simulink model "simulation_darko_vol_ligne"  (R2021b)
settings: Solver=ode23s  StartTime=0.0  StopTime=60  FixedStep=0.0001  MaxStep=1e-2  RelTol=1e-3
values from neighbouring files (symbols this model uses):
  controlleur = struct('k1',1.0,                       'kc',5,                       'kv',1.0,                       'ku',600.0,                       'kgamma',1.0,                       'M_k',M_k,                       'kd',60,                       'k_s',0.01                       )    [generateContolleur.m]    (also in run_vol_ligne.m = generateContolleur(drone))
  drone = generateDarko()    [jacobian.m]    (also in run_vol_ligne.m)
  initial_state = [p_initial; v_initial; q_initial; omega_initial]    [run_vol_ligne.m]
  p2 = [1000; 1000; 1000]    [run_vol_ligne.m]
  speed = 20    [run_vol_ligne.m]
libraries: simulink_extras x6, aerolibanim x1, slpidlib x1, sharedtransform x1
settings Model: Creator=florian  LastModifiedBy=florian
settings SolverCC: AlgebraicLoopSolver=TrustRegion
settings DebuggingCC: SFMachineParentedDataDiag=warning

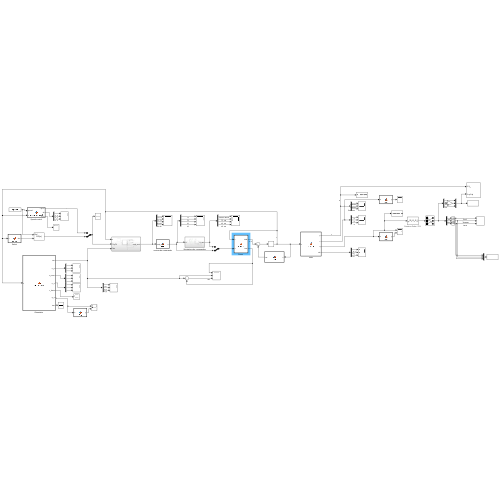
[thumbnail: Simulink's stored preview of the top-level diagram]
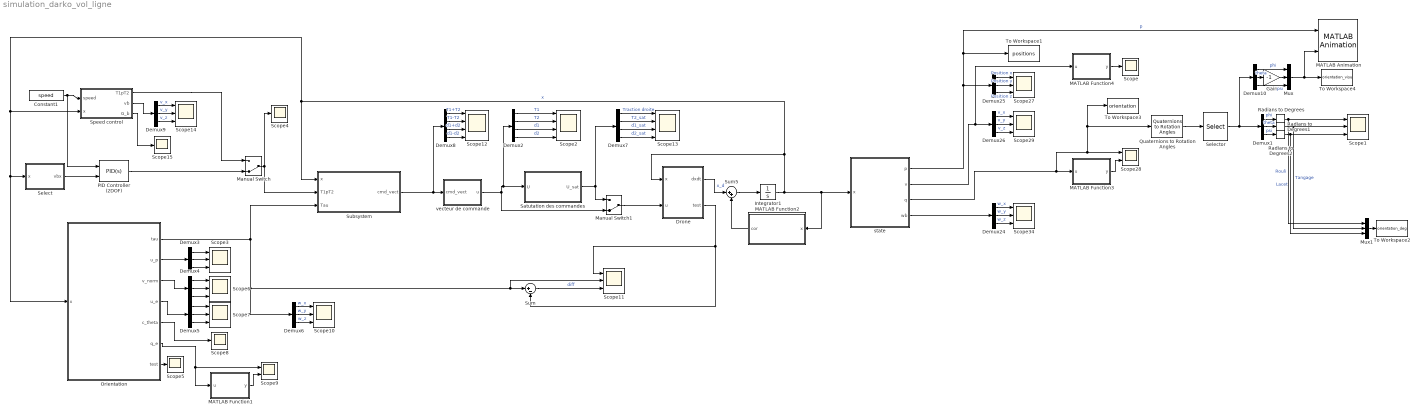
== system simulation_darko_vol_ligne ==
  Constant1 : Constant  Value=speed
  Demux{1,3..6,9..10,24..26} (10 alike) : Demux  Outputs=3
  Demux2 : Demux
  Demux7 : Demux
  Demux8 : Demux
  Drone : MATLAB Function  TreatAsAtomicUnit=on
  Gain : Gain  Gain=-1
  Integrator1 : Integrator  InitialCondition=initial_state
  MATLAB Animation : aerolibanim/MATLAB Animation  Tag=Matlab Animation 6 DOF  Vehicles=1  Geometries='astredwedge.mat'  BoundingBoxCoordinates=[-50,50,-50,50,-50,50]  CameraOffset=[-150,-50,0]  CameraViewAngle=3  SampleTime=0.2  FigurePosition=[962,411,639,384]
      settings: SourceProductBaseCode=AE
  MATLAB Function1 : MATLAB Function  TreatAsAtomicUnit=on
  MATLAB Function2 : MATLAB Function  TreatAsAtomicUnit=on
  MATLAB Function3 : MATLAB Function  TreatAsAtomicUnit=on
  MATLAB Function4 : MATLAB Function  TreatAsAtomicUnit=on
  Manual Switch : ManualSwitch  CurrentSetting=0
  Manual Switch1 : ManualSwitch  CurrentSetting=0
  Mux : Mux  Inputs=3
  Mux1 : Mux  Inputs=3
  Orientation : MATLAB Function  TreatAsAtomicUnit=on
  PID Controller (2DOF) : slpidlib/PID Controller (2DOF)  Controller=PID  Form=Parallel  TimeDomain=Continuous-time  UseExternalTs=off  SampleTime=-1  IntegratorMethod=Forward Euler  FilterMethod=Forward Euler  ControllerParametersSource=internal  P=1  I=1  D=0.1  UseFilter=on  N=100  b=1  c=1  TunerSelectOption=Transfer Function Based (PID Tuner App)  InitialConditionSource=internal  InitialConditionForIntegrator=0  InitialConditionForFilter=0  DifferentiatorICPrevScaledInput=0  ExternalReset=none  TrackingMode=off  Kt=1  LimitOutput=off  SatLimitsSource=internal  UpperSaturationLimit=inf  LowerSaturationLimit=-inf  LinearizeAsGain=on  AntiWindupMode=none  Kb=1  POutMin=[]  POutMax=[]  IOutMin=[]  IOutMax=[]  DOutMin=[]  DOutMax=[]  NOutMin=[]  NOutMax=[]  bOutMin=[]  bOutMax=[]  cOutMin=[]  cOutMax=[]  SumOutMin=[]  SumOutMax=[]  SaturationOutMin=[]  SaturationOutMax=[]  PParamMin=[]  PParamMax=[]  IParamMin=[]  IParamMax=[]  DParamMin=[]  DParamMax=[]  NParamMin=[]  NParamMax=[]  bParamMin=[]  bParamMax=[]  cParamMin=[]  cParamMax=[]  KbParamMin=[]  KbParamMax=[]  KtParamMin=[]  KtParamMax=[]  KbOutMin=[]  KbOutMax=[]  KtOutMin=[]  KtOutMax=[]  IntegratorOutMin=[]  IntegratorOutMax=[]  FilterOutMin=[]  FilterOutMax=[]  SumI1OutMin=[]  SumI1OutMax=[]  SumI2OutMin=[]  SumI2OutMax=[]  SumI3OutMin=[]  SumI3OutMax=[]  SumI4OutMin=[]  SumI4OutMax=[]  SumDOutMin=[]  SumDOutMax=[]  Sum1OutMin=[]  Sum1OutMax=[]  Sum2OutMin=[]  Sum2OutMax=[]  Sum3OutMin=[]  Sum3OutMax=[]  DifferentiatorOutMin=[]  DifferentiatorOutMax=[]  FilterDiffOutCoefMin=[]  FilterDiffOutCoefMax=[]  ReciprocalOutMin=[]  ReciprocalOutMax=[]  SumDenOutMin=[]  SumDenOutMax=[]  SumNumOutMin=[]  SumNumOutMax=[]  DivideOutMin=[]  DivideOutMax=[]  UdiffTsProdOutMin=[]  UdiffTsProdOutMax=[]  NTsProdOutMin=[]  NTsProdOutMax=[]  UintegralTsProdOutMin=[]  UintegralTsProdOutMax=[]  UngainTsProdOutMin=[]  UngainTsProdOutMax=[]  IntegratorContinuousStateAttributes=''  IntegratorStateMustResolveToSignalObject=off  IntegratorRTWStateStorageClass=Auto  FilterContinuousStateAttributes=''  FilterStateMustResolveToSignalObject=off  FilterRTWStateStorageClass=Auto  ParallelPVariant=InternalParameters  IdealPVariant=Disabled  IVariant=InternalParameters  DVariant=InternalParameters  bVariant=InternalParameters  cVariant=InternalParameters  IntegratorVariant=Continuous  SatVariant=Disabled  AWVariant=Passthrough  PCopyVariant=Disabled  TRVariant=Disabled  FdbkBlocksVariant=Forward  IdealPFdbkVariant=Disabled  SatFdbkVariant=Disabled  DerivativeFilterVariant=ContFilter  NVariant=InternalParameters  NCopyVariant=Disabled  FilterICVariant=InternalICsFilter  IntegratorICVariant=InternalICs  ExternalResetVariant=Disabled  TRSumVariant=Passthrough  SumFdbkVariant=Disabled  SumVariant=Sum_PID  TsampFilterVariant=InternalTs  TsampNgainVariant=Passthrough  TsampIntegralVariant=Passthrough  ExternalSaturationOutDataTypeStr=Inherit: Same as second input
      settings: SourceProductBaseCode=SL
  Quaternions to Rotation Angles : sharedtransform/Quaternions to Rotation Angles  rotationOrder=ZXY  aMode=aMode
      settings: SourceProductBaseCode=AE,PW,DR,MT,UV,VE
  Radians to Degrees : simulink_extras/Transformations/Radians to Degrees
  Radians to Degrees1 : simulink_extras/Transformations/Radians to Degrees
  Radians to Degrees2 : simulink_extras/Transformations/Radians to Degrees
  Satutation des commandes : Subsystem
  Scope{,4..5,8,15} (5 alike) : Scope
  Scope{1,3,6..7,10..11,14,27,29,34} (10 alike) : Scope  NumInputPorts=3
  Scope12 : Scope  NumInputPorts=4
  Scope13 : Scope  NumInputPorts=4
  Scope2 : Scope  NumInputPorts=4
  Scope28 : Scope  NumInputPorts=2
  Scope9 : Scope  NumInputPorts=2
  Select : MATLAB Function  TreatAsAtomicUnit=on
  Selector : Selector  InputPortWidth=3  IndexOptions=Index vector (dialog)  Indices=[2 3 1]  OutputSizes=1
  Speed control : MATLAB Function  TreatAsAtomicUnit=on
  Subsystem : Subsystem
  Sum : Sum  Inputs=|+-
  Sum5 : Sum  Inputs=|++
  To Workspace1 : ToWorkspace  VariableName=positions  SampleTime=-1
  To Workspace2 : ToWorkspace  VariableName=orientation_deg  SampleTime=-1
  To Workspace3 : ToWorkspace  VariableName=orientation  SampleTime=-1
  To Workspace4 : ToWorkspace  VariableName=orientation_visu  SampleTime=-1
  state : MATLAB Function  TreatAsAtomicUnit=on
  vecteur de commande : MATLAB Function  TreatAsAtomicUnit=on
  wires:
  Demux24/1 -> Scope34/1  "w_x"
  MATLAB Function3/1(y) -> Scope28/2
  Drone/1(dxdt) -> Sum5/1  "x_d"
  Demux24/2 -> Scope34/2  "w_y"
  Demux25/2 -> Scope27/2  "Position y"
  Integrator1/1 -> Drone/1(x), Select/1(x), Orientation/1(x), Speed control/2(x), Subsystem/1(x), MATLAB Function2/1(x), state/1(x)  "x"
  state/3(q) -> Scope28/1, To Workspace3/1, Quaternions to Rotation Angles/1, MATLAB Function3/1(u)
  Sum5/1 -> Integrator1/1
  MATLAB Function2/1(cor) -> Sum5/2
  Demux26/3 -> Scope29/3  "v_z"
  Demux26/2 -> Scope29/2  "v_y"
  Demux25/1 -> Scope27/1  "Position x"
  Demux25/3 -> Scope27/3  "Position z"
  state/1(p) -> MATLAB Animation/1, To Workspace1/1, Demux25/1  "p"
  Demux24/3 -> Scope34/3  "w_z"
  Demux26/1 -> Scope29/1  "v_x"
  Quaternions to Rotation Angles/1 -> Selector/1
  Satutation des commandes/1(U_sat) -> Demux7/1, Manual Switch1/1
  state/2(v) -> MATLAB Function4/1(u), Demux26/1
  Constant1/1 -> PID Controller (2DOF)/1, Speed control/1(speed)
  state/4(wb) -> Demux24/1
  Demux1/3 -> Radians to Degrees2/1  "psi"
  Demux1/2 -> Radians to Degrees1/1  "theta"
  Demux1/1 -> Radians to Degrees/1  "phi"
  Selector/1 -> Demux10/1, Demux1/1
  vecteur de commande/1(u) -> Demux2/1, Satutation des commandes/1(U), Manual Switch1/2
  Manual Switch1/1 -> Drone/2(u)
  Demux3/3 -> Scope3/3
  Demux3/1 -> Scope3/1
  Orientation/2(u_p) -> Demux3/1
  Demux3/2 -> Scope3/2
  Demux4/3 -> Scope6/3
  Demux4/1 -> Scope6/1
  Orientation/3(v_norm) -> Demux4/1
  Demux4/2 -> Scope6/2
  Orientation/4(u_e) -> Demux5/1
  Demux5/3 -> Scope7/3
  Demux5/2 -> Scope7/2
  Demux5/1 -> Scope7/1
  Orientation/5(c_theta) -> Scope8/1
  MATLAB Function1/1(y) -> Scope9/2
  Orientation/6(q_e) -> MATLAB Function1/1(u), Scope9/1
  Demux6/3 -> Scope10/3  "w_z"
  Demux6/1 -> Scope10/1  "w_x"
  Demux6/2 -> Scope10/2  "w_y"
  Sum/1 -> Scope11/3  "diff"
  Demux8/1 -> Scope12/1  "T1+T2"
  Demux8/2 -> Scope12/2  "T1-T2"
  Demux8/3 -> Scope12/3  "d1+d2"
  Demux8/4 -> Scope12/4  "d1-d2"
  Demux2/1 -> Scope2/1  "T1"
  Demux2/4 -> Scope2/4  "d2"
  Demux2/3 -> Scope2/3  "d1"
  Demux2/2 -> Scope2/2  "T2"
  Demux7/1 -> Scope13/1  "Traction droite"
  Demux7/4 -> Scope13/4  "d2_sat"
  Demux7/3 -> Scope13/3  "d1_sat"
  Demux7/2 -> Scope13/2  "T2_sat"
  Demux9/1 -> Scope14/1  "v_x"
  Speed control/2(vb) -> Demux9/1
  Demux9/3 -> Scope14/3  "v_z"
  Demux9/2 -> Scope14/2  "v_y"
  Speed control/3(G_b) -> Scope15/1
  Drone/2(test) -> Sum/2, Scope11/1
  Speed control/1(T1pT2) -> Manual Switch/1
  PID Controller (2DOF)/1 -> Manual Switch/2
  Select/1(vbx) -> PID Controller (2DOF)/2
  Manual Switch/1 -> Scope4/1, Subsystem/2(T1pT2)
  Orientation/7(test) -> Scope5/1
  Mux1/1 -> To Workspace2/1
  Radians to Degrees/1 -> Mux1/1, Scope1/1  "Rouli"
  Radians to Degrees2/1 -> Mux1/3, Scope1/3  "Lacet"
  Radians to Degrees1/1 -> Mux1/2, Scope1/2  "Tangage"
  MATLAB Function4/1(y) -> Scope/1
  Subsystem/1(cmd_vect) -> Demux8/1, vecteur de commande/1(cmd_vect)
  Orientation/1(tau) -> Subsystem/3(Tau), Scope11/2, Sum/1, Demux6/1
  Demux10/1 -> Mux/1  "phi"
  Demux10/2 -> Gain/1  "theta"
  Gain/1 -> Mux/2
  Demux10/3 -> Mux/3  "psi"
  Mux/1 -> To Workspace4/1, MATLAB Animation/2

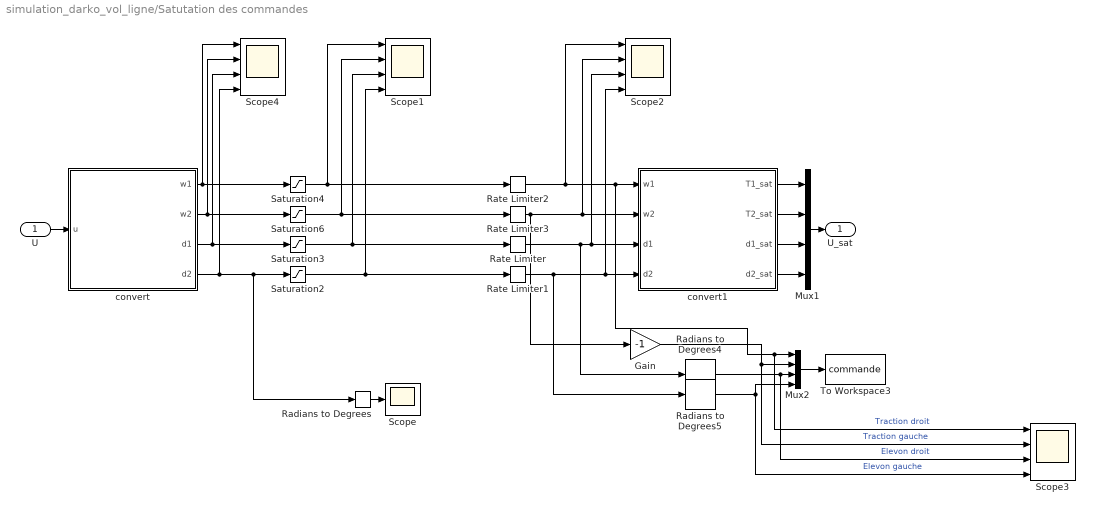
== system simulation_darko_vol_ligne/Satutation des commandes ==
  U : Inport
  Gain : Gain  Gain=-1
  Mux1 : Mux
  Mux2 : Mux
  Radians to Degrees : simulink_extras/Transformations/Radians to Degrees
  Radians to Degrees4 : simulink_extras/Transformations/Radians to Degrees
  Radians to Degrees5 : simulink_extras/Transformations/Radians to Degrees
  Rate Limiter : RateLimiter  RisingSlewLimit=drone.ELEVON_RATE_CHANGE  FallingSlewLimit=-drone.ELEVON_RATE_CHANGE  SampleTimeMode=inherited
  Rate Limiter1 : RateLimiter  RisingSlewLimit=drone.ELEVON_RATE_CHANGE  FallingSlewLimit=-drone.ELEVON_RATE_CHANGE  SampleTimeMode=inherited
  Rate Limiter2 : RateLimiter  RisingSlewLimit=drone.MOTOR_RATE_CHANGE  FallingSlewLimit=-drone.MOTOR_RATE_CHANGE  SampleTimeMode=inherited
  Rate Limiter3 : RateLimiter  RisingSlewLimit=drone.MOTOR_RATE_CHANGE  FallingSlewLimit=-drone.MOTOR_RATE_CHANGE  SampleTimeMode=inherited
  Saturation2 : Saturate  UpperLimit=30*(pi/180)  LowerLimit=-30*(pi/180)
  Saturation3 : Saturate  UpperLimit=30*(pi/180)  LowerLimit=-30*(pi/180)
  Saturation4 : Saturate  UpperLimit=1000  LowerLimit=200
  Saturation6 : Saturate  UpperLimit=1000  LowerLimit=200
  Scope : Scope
  Scope{1..4} (4 alike) : Scope  NumInputPorts=4
  To Workspace3 : ToWorkspace  VariableName=commande  SampleTime=-1
  convert : MATLAB Function  TreatAsAtomicUnit=on
  convert1 : MATLAB Function  TreatAsAtomicUnit=on
  U_sat : Outport
  wires:
  convert/1(w1) -> Saturation4/1, Scope4/1
  convert/2(w2) -> Scope4/2, Saturation6/1
  convert/3(d1) -> Scope4/3, Saturation3/1
  convert1/1(T1_sat) -> Mux1/1
  convert1/4(d2_sat) -> Mux1/4
  Mux1/1 -> U_sat/1
  convert1/2(T2_sat) -> Mux1/2
  convert1/3(d1_sat) -> Mux1/3
  Saturation6/1 -> Rate Limiter3/1, Scope1/2
  Saturation4/1 -> Rate Limiter2/1, Scope1/1
  U/1 -> convert/1(u)
  Saturation3/1 -> Rate Limiter/1, Scope1/3
  Saturation2/1 -> Rate Limiter1/1, Scope1/4
  convert/4(d2) -> Radians to Degrees/1, Saturation2/1, Scope4/4
  Radians to Degrees/1 -> Scope/1
  Rate Limiter/1 -> Radians to Degrees4/1, Scope2/3, convert1/3(d1)
  Radians to Degrees5/1 -> Mux2/4, Scope3/4  "Elevon gauche"
  Radians to Degrees4/1 -> Scope3/3, Mux2/3  "Elevon droit"
  Rate Limiter2/1 -> Scope2/1, Scope3/1, Mux2/1, convert1/1(w1)  "Traction droit"
  Rate Limiter1/1 -> Radians to Degrees5/1, Scope2/4, convert1/4(d2)
  Rate Limiter3/1 -> Gain/1, Scope2/2, convert1/2(w2)
  Gain/1 -> Scope3/2, Mux2/2  "Traction gauche"
  Mux2/1 -> To Workspace3/1

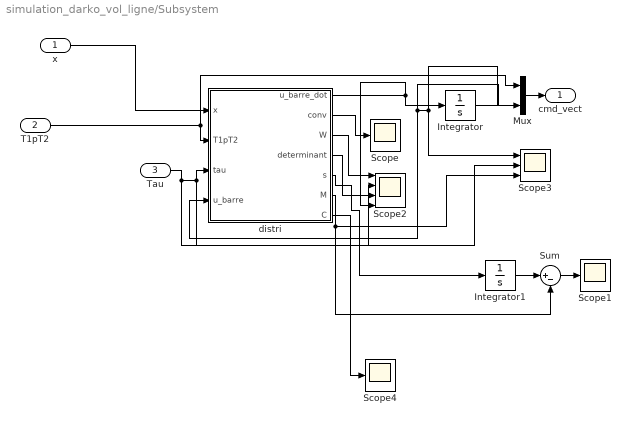
== system simulation_darko_vol_ligne/Subsystem ==
  x : Inport
  T1pT2 : Inport  Port=2
  Tau : Inport  Port=3
  Integrator : Integrator  InitialCondition=[0;0;0]
  Integrator1 : Integrator
  Mux : Mux  Inputs=2
  Scope : Scope
  Scope1 : Scope
  Scope2 : Scope  NumInputPorts=4
  Scope3 : Scope  NumInputPorts=3
  Scope4 : Scope
  Sum : Sum  Inputs=|+-
  distri : MATLAB Function  TreatAsAtomicUnit=on
  cmd_vect : Outport
  wires:
  Integrator/1 -> distri/4(u_barre), Scope3/1, Mux/2
  Mux/1 -> cmd_vect/1
  distri/2(conv) -> Scope/1
  distri/4(determinant) -> Scope2/3
  distri/3(W) -> Scope2/1
  distri/5(s) -> Integrator1/1
  Integrator1/1 -> Sum/1
  distri/6(M) -> Sum/2, Scope3/3
  Sum/1 -> Scope1/1
  x/1 -> distri/1(x)
  T1pT2/1 -> distri/2(T1pT2), Mux/1
  Tau/1 -> Scope3/2, Scope2/2, distri/3(tau)
  distri/1(u_barre_dot) -> Integrator/1, Scope2/4
  distri/7(C) -> Scope4/1

== matlab function simulation_darko_vol_ligne/Select ==
  data: x input; vbx output
function vbx = select(x)
v = x(4:6);
q  = x(7:10);
D = q2dcm(q);

vb = D'*v;
vbx = vb(1);

== matlab function simulation_darko_vol_ligne/MATLAB Function4 ==
  data: u input; y output
function y = fcn(u)
%#codegen

y = norm(u);

== matlab function simulation_darko_vol_ligne/Satutation des commandes/convert ==
  data: u input size=4; w1 output; drone parameter; w2 output; d1 output; d2 output
function [w1, w2, d1, d2] = convert(u, drone)
%#codegen
kf = drone.PROP_KP;

T1 = max(u(1),0);
T2 = max(u(2),0);
d1 = u(3);
d2 = u(4);

w1 = sqrt(T1/kf);
w2 = sqrt(T2/kf);

== matlab function simulation_darko_vol_ligne/Satutation des commandes/convert1 ==
  data: w1 input; w2 input; d1 input; d2 input; T1_sat output; T2_sat output; drone parameter; d1_sat output; d2_sat output
function [T1_sat, T2_sat, d1_sat, d2_sat] = convert2(w1, w2, d1, d2, drone)
%#codegen
kf = drone.PROP_KP;

T1_sat = kf*w1^2;
d1_sat = d1;
T2_sat = kf*w2^2;
d2_sat = d2;

== matlab function simulation_darko_vol_ligne/MATLAB Function2 ==
  data: x input; cor output
function cor  = fcn(x)
%#codegen
q  = x(7:10);
n = norm(q);
mismatch = 1-n;
cor = [0;0;0; 0;0;0; mismatch*q; 0;0;0];

== matlab function simulation_darko_vol_ligne/MATLAB Function3 ==
  data: u input; y output
function y = fcn(u)
%#codegen

y = norm(u);

== matlab function simulation_darko_vol_ligne/state ==
  data: x input; p output; v output; q output; wb output
function [p, v,q, wb] = demux(x)
%#codegen

p = x(1:3);
v = x(4:6);
q  = x(7:10);
wb = x(11:13);

== matlab function simulation_darko_vol_ligne/Subsystem/distri ==
  data: x input; T1pT2 input; tau input; u_barre input; u_barre_dot output; controlleur parameter; drone parameter; conv output; W output; determinant output; s output; M output; C output
function [u_barre_dot, conv,W, determinant, s, M, C]= dist(x, T1pT2, tau, u_barre, controlleur, drone)

% p = x(1:3);
v = x(4:6);
q  = x(7:10);
w = x(11:13);

T1mT2 = u_barre(1);
d1pd2 = u_barre(2);
d1md2 = u_barre(3);


D = q2dcm(q);

%% velocityin body frame
vb = D'*v;
vbx = vb(1);
vby = vb(2);
vbz = vb(3);

J = drone.INERTIA;


ay = drone.P_A2_CG(2);
py = drone.P_P2_CG(2);
die_c = drone.PHI(3,3);
Cd0 = drone.PHI(1,1);

Swet   = drone.WET_SURFACE;
Sdry   = drone.DRY_SURFACE;
Sp = pi*drone.PROP_RADIUS^2;
Thetam = drone.ELEVON_MEFFICIENCY(2);
Thetaf = drone.ELEVON_FEFFICIENCY(2);
kf = drone.PROP_KP;
km = drone.PROP_KM;
S = Swet + Sdry;
rho    = drone.RHO;
phi_n  = drone.PHI_n;
chord  = drone.CHORD;
ws     = drone.WINGSPAN;
B = diag([ws; chord; ws]);
dR = drone.CENTRAGE ;

eta = sqrt( norm(v)^2 + phi_n*norm(B*w)^2 );

% M = [
% (km/kf - (Swet/(8*Sp)) * ay * die_c * Thetaf *d1pd2)*T1mT2 + (-(Swet/(8*Sp))* ay * die_c * Thetaf* T1pT2 + 1/4 * rho* S * eta * ay * die_c * Thetaf* vbx)*d1md2; 
% (Swet/(8*Sp) * dR * die_c * Thetam * T1pT2 + 1/4 * rho* S * eta * dR * die_c * Thetam* vbx )* d1pd2 + Swet/(8*Sp) * dR * die_c * Thetam * T1mT2*d1md2 + 1/2 * rho* S *  dR  * die_c * eta *vbz ;
% -(py+Swet/(4*Sp)*ay*Cd0)*T1mT2 + (1/4 * rho* S * eta * ay * Cd0 * Thetaf* vbz)*d1md2
%     ];

x= T1mT2 ;
y = d1pd2;
z = d1md2;

M = [
(km/kf - (Swet/(8*Sp)) * ay * die_c * Thetaf *y)*x + (-(Swet/(8*Sp))* ay * die_c * Thetaf* T1pT2 + 1/4 * rho* S * eta * ay * die_c * Thetaf* vbx)*z; 
(Swet/(8*Sp) * dR * die_c * Thetam * T1pT2 + 1/4 * rho* S * eta * dR * die_c * Thetam* vbx )* y + Swet/(8*Sp) * dR * die_c * Thetam * x*z + 1/2 * rho* S *  dR  * die_c * eta *vbz ;
-(py+Swet/(4*Sp)*ay*Cd0)*x + (1/4 * rho* S * eta * ay * Cd0 * Thetaf* vbz)*z
    ];

% M =J*M;
 
dM = [km/kf - (Swet/(8*Sp)) * ay * die_c * Thetaf *d1pd2, -(Swet/(8*Sp))* ay * die_c * Thetaf * T1mT2 ,(-(Swet/(8*Sp))* ay * die_c * Thetaf* T1pT2 + 1/4 * rho* S * eta * ay * die_c * Thetaf* vbx);
(Swet/(8*Sp) * dR * die_c * Thetam * d1md2), Swet/(8*Sp) * dR * die_c * Thetam * T1pT2 + 1/4 * rho* S * eta * dR * die_c * Thetam* vbx, Swet/(8*Sp) * dR * die_c * Thetam * T1mT2;
-(py+Swet/(4*Sp)*ay*Cd0), 0, 1/4 * rho* S * eta * ay * Cd0 * Thetaf* vbz
     ];
% dM = J*dM;

sat_val = 10000;
[U,S,V] = svd(dM);
C = cond(dM);

inv_S = zeros(3);
inv_S(1,1) = min(sat_val, max(-sat_val, 1/S(1,1)));
inv_S(2,2) = min(sat_val, max(-sat_val, 1/S(2,2)));
inv_S(3,3) = min(sat_val, max(-sat_val, 1/S(3,3)));

% inv_dM = V*inv(S)*U';
inv_dM = V*inv_S*U';

% u_barre_dot = - controlleur.ku * inv(dM)*(M - tau );
u_barre_dot = - controlleur.ku * inv_dM*(M - tau );
% u_barre_dot = - 0.01 * dM*(M - tau );

conv= M - tau ;
W = (M - tau)'*(M - tau);
determinant = det(dM);
s = dM*u_barre_dot;

== matlab function simulation_darko_vol_ligne/Drone ==
  data: x input; u input; dxdt output; drone parameter; test output
function [dxdt,test] = drone(x, u, drone)

%% physical constants
% gravity
g = drone.G;
% vehicle mass
m = drone.MASS;
% vehicle inertia matrix
J = drone.INERTIA; % [3x3 real symmetric] in body axis

%% state demultiplexing
% p = x(1:3);
v = x(4:6);
q  = x(7:10);
wb = x(11:13);

Rq = q2dcm(q);

[Fp, Mp] = external_force_moment(x, u, 0, drone);

T1 = u(1);
T2 = u(2);
d1 = u(3);
d2 = u(4);

u_prime = [T1;T2;T1*d1; T2*d2];
% position
dpdt = v;

% kinematics
dvdt =  -Rq'*[0;0;g] + (1/m)*drone.Fb*u_prime + (1/m)*Fp; 


%% quaternion derivative
eta = q(1);
eps = q(2:4);

dqdt = (1/2)*[-eps'; eta*eye(3) + skew_sym(eps)]*wb;

%% angular velocity derivative
% kinematics
dwdt = -J\cross(wb, J*wb) + J\(drone.Mb*u_prime) + J\Mp;
test = (drone.Mb*u_prime)+Mp;

%% derivative multiplexing
dxdt = [dpdt; dvdt; dqdt; dwdt] ;

== matlab function simulation_darko_vol_ligne/Speed control ==
  data: speed input; x input; T1pT2 output; controlleur parameter; drone parameter; vb output; G_b output
function [T1pT2, vb, G_b]   = speed_control(speed, x, controlleur, drone)
%#codegen 

% gravity
g = drone.G;
% vehicle mass
m = drone.MASS;
rho = drone.RHO;
% ws = drone.WINGSPAN;
% chord = drone.CHORD;
Swet = drone.WET_SURFACE;
Sdry = drone.DRY_SURFACE;
S = Swet + Sdry;

PHI_fv = drone.PHI(1:3,1:3);


% p = x(1:3);
v = x(4:6);
q  = x(7:10);
w = x(11:13);

eta = sqrt(norm(v)^2);
D = q2dcm(q);

vb = D'*v;
vbx = vb(1);
% vby = vb(2);
% vbz = vb(3);

G_b = D'*[0;0;g];

ay = drone.P_A2_CG(2);
py = drone.P_P2_CG(2);
die_c = drone.PHI(3,3);
Cd0 = drone.PHI(1,1);

Swet   = drone.WET_SURFACE;
Sdry   = drone.DRY_SURFACE;
Sp = pi*drone.PROP_RADIUS^2;
Thetam = drone.ELEVON_MEFFICIENCY(2);
% Thetaf = drone.ELEVON_FEFFICIENCY(2);
kf = drone.PROP_KP;
km = drone.PROP_KM;
S = Swet + Sdry;
rho    = drone.RHO;
phi_n  = drone.PHI_n;
chord  = drone.CHORD;
ws     = drone.WINGSPAN;
B = diag([ws; chord; ws]);
dR = drone.CENTRAGE ;
eta = sqrt( norm(v)^2 + phi_n*norm(B*w)^2 );

% T1pT2 = 1/(2*(1-(Swet/(4*Sp))*Cd0))*rho*S*eta*Cd0*vbx + G_b(1) + controlleur.kv * (speed - vb(1));
 T1pT2 = controlleur.kv * (speed - vb(1));

== matlab function simulation_darko_vol_ligne/MATLAB Function1 ==
  data: u input; y output
function y = fcn(u)
%#codegen

% y = norm(u);
y = sqrt(u'*u);

== matlab function simulation_darko_vol_ligne/vecteur de commande ==
  data: cmd_vect input; u output
function u = fcn(cmd_vect)

T1pT2 = cmd_vect(1);
T1mT2 = cmd_vect(2);
d1pd2 = cmd_vect(3);
d1md2 = cmd_vect(4);

u = [1/2*(T1pT2 + T1mT2); 1/2*(T1pT2 - T1mT2); 1/2*(d1pd2 + d1md2); 1/2*(d1pd2 - d1md2)];

== matlab function simulation_darko_vol_ligne/Orientation ==
  data: tau output; u_p output; v_norm output; x input; p2 parameter; controlleur parameter; drone parameter; u_e output; c_theta output; q_e output; test output
function [tau, u_p, v_norm, u_e, c_theta, q_e, test]= orientation(x, p2, controlleur, drone)
%#codegen
p = x(1:3);
v = x(4:6);
% q  = x(7:10);
wb = x(11:13);

J = drone.INERTIA;


u_p = (p2-p)/norm(p2-p);
v_norm = v/norm(v);



c_theta = u_p'*v_norm;      %cos (theta)
% theta = acos(c_theta);
u_e = cross(u_p, v_norm); 
test = norm(u_e);

% q_e = [c_theta; u_e];



if(norm(u_e) ~= 0)
    q_e = [sqrt((1+c_theta)/2); (u_e / norm(u_e))*sqrt((1-c_theta)/2)];
%     q_e = [cos(theta/2);(u_e / norm(u_e))*sin(theta/2)];
else
    q_e = [1;0;0;0];
end

tau = -controlleur.kc*sign(q_e(1))*q_e(2:4) + cross(wb, J*wb) - controlleur.kd * wb;

% gain = diag([0.05;0.5;0.005]);
% tau = -gain*sign(q_e(1))*q_e(2:4);

% tau = -controlleur.kc*q_e(1)*q_e(2:4) + cross(wb, J*wb);
